simulink model "ElbowMusculoSkeletalModel"  (R2022b)
settings: Solver=FixedStepAuto  StartTime=0.0  StopTime=10  FixedStep=tstep  RelTol=1e-3
model workspace: external: MATLAB File C:\Users\hp\Desktop\Study\RAS MAE\EEE587\Project\ActivationDynamicsParameters.m (data not in the file)
values from neighbouring files (symbols this model uses):
  a0 = 0.286    [AllMuscleParams.m]    (also in equations.m)
  a1e = -0.014    [AllMuscleParams.m]    (also in equations.m)
  a2e = -3.96e-3    (= -0.00396)    [AllMuscleParams.m]    (also in equations.m)
  arel = 0.41    [AllMuscleParams.m]    (also in equations.m)
  brel = 5.2    [AllMuscleParams.m]    (also in equations.m)
  c = 1.373e-4    (= 0.0001373)    [AllMuscleParams.m]    (also in equations.m)
  Fmax = 1420    [AllMuscleParams.m]    (also in equations.m)
  Iarm = Marm*(Llarm^2)/3    (= 0.208333333333)    [AllMuscleParams.m]    (also in equations.m = Marm*(Llarm^2)/3)
  k = 2.90    (= 2.9)    [AllMuscleParams.m]    (also in equations.m)
  kpe = (0.5*Fmax)/(1 + width - (lpe_0/lce_opt))    (= 2730.76923077)    [AllMuscleParams.m]
  kse = Fmax/((0.04*lse_0)^2)    (= 29999323.9589)    [AllMuscleParams.m]    (also in equations.m = Fmax/((0.04*lse_0)^2))
  lce_init = lmtc_init-lse_0    (= 0.114)    [AllMuscleParams.m]
  lce_opt = 0.092    [AllMuscleParams.m]    (also in equations.m)
  Llarm = 0.5    [AllMuscleParams.m]    (also in equations.m)
  lpe_0 = 1.4*lce_opt    (= 0.1288)    [AllMuscleParams.m]
  lse_0 = 0.172    [AllMuscleParams.m]    (also in equations.m)
  m = 11.25    [AllMuscleParams.m]    (also in equations.m)
  Marm = 2.5    [AllMuscleParams.m]    (also in equations.m)
  q0 = 0.005    [AllMuscleParams.m]    (also in equations.m)
  qcrit = 0.03    [AllMuscleParams.m]
  ThetaInit = 0    [AllMuscleParams.m]
undefined symbols (not defined in the file or in its folder): DiscIntNeverNeededParam
libraries: simulink x2
settings Model: Creator=hp  LastModifiedBy=hp

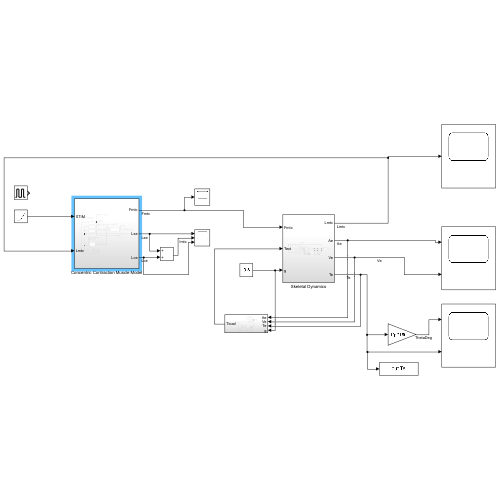
[thumbnail: Simulink's stored preview of the top-level diagram]
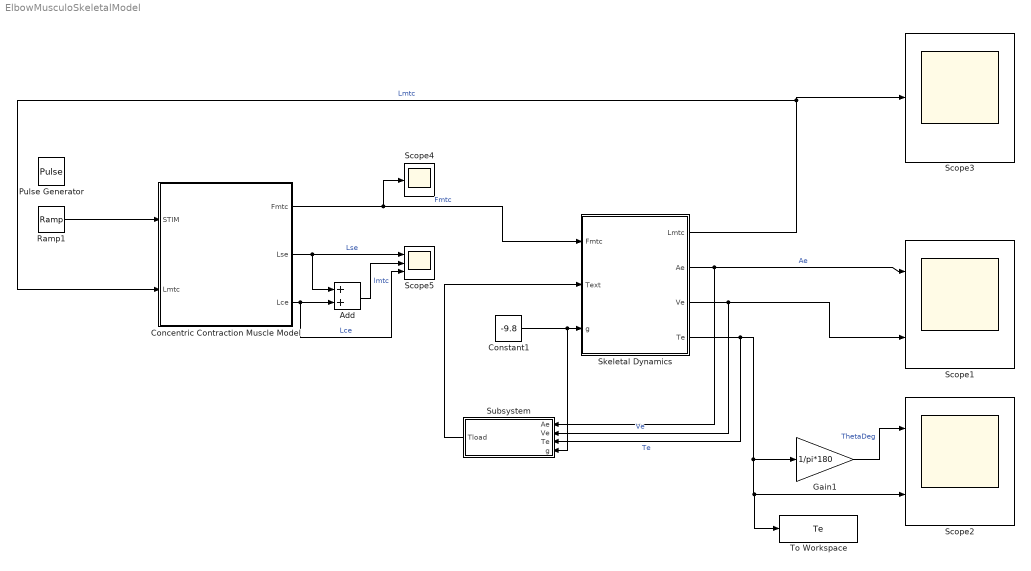
== system ElbowMusculoSkeletalModel ==
  Add : Sum
  Concentric Contraction Muscle Model : Subsystem
  Constant1 : Constant  Value=-9.8
  Gain1 : Gain  Gain=1/pi*180
  Pulse Generator : DiscretePulseGenerator  PulseType=Time based  Amplitude=10  Period=0.01  PulseWidth=50
  Ramp1 : simulink/Sources/Ramp  slope=0  start=0  InitialOutput=0.1
  Scope1 : Scope  NumInputPorts=2
  Scope2 : Scope  NumInputPorts=2
  Scope3 : Scope
  Scope4 : Scope
  Scope5 : Scope  NumInputPorts=3
  Skeletal Dynamics : Subsystem
  Subsystem : Subsystem
  To Workspace : ToWorkspace  VariableName=Te  SaveFormat=Timeseries  SampleTime=-1
  wires:
  Constant1/1 -> Subsystem/4(g), Skeletal Dynamics/3(g)
  Skeletal Dynamics/3(Ve) -> Subsystem/2(Ve), Scope1/2  "Ve"
  Skeletal Dynamics/4(Te) -> Subsystem/3(Te), To Workspace/1, Scope2/2, Gain1/1  "Te"
  Gain1/1 -> Scope2/1  "ThetaDeg"
  Skeletal Dynamics/2(Ae) -> Subsystem/1(Ae), Scope1/1  "Ae"
  Skeletal Dynamics/1(Lmtc) -> Concentric Contraction Muscle Model/2(Lmtc), Scope3/1  "Lmtc"
  Concentric Contraction Muscle Model/1(Fmtc) -> Skeletal Dynamics/1(Fmtc), Scope4/1  "Fmtc"
  Concentric Contraction Muscle Model/2(Lse) -> Add/1, Scope5/1  "Lse"
  Concentric Contraction Muscle Model/3(Lce) -> Add/2, Scope5/3  "Lce"
  Add/1 -> Scope5/2  "lmtc"
  Subsystem/1(Tload) -> Skeletal Dynamics/2(Text)
  Ramp1/1 -> Concentric Contraction Muscle Model/1(STIM)

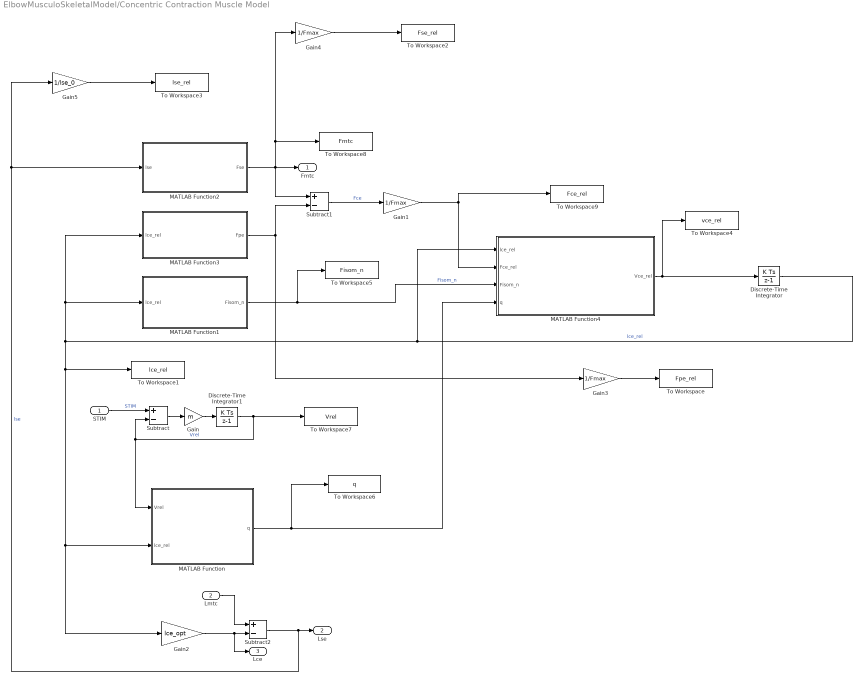
== system ElbowMusculoSkeletalModel/Concentric Contraction Muscle Model ==
  STIM : Inport
  Lmtc : Inport  Port=2
  Discrete-Time Integrator : DiscreteIntegrator  InitialCondition=lce_init/lce_opt  SampleTime=-1  ICPrevOutput=DiscIntNeverNeededParam  ICPrevScaledInput=DiscIntNeverNeededParam
  Discrete-Time Integrator1 : DiscreteIntegrator  SampleTime=-1  ICPrevOutput=DiscIntNeverNeededParam  ICPrevScaledInput=DiscIntNeverNeededParam
  Gain : Gain  Gain=m
  Gain1 : Gain  Gain=1/Fmax
  Gain2 : Gain  Gain=lce_opt
  Gain3 : Gain  Gain=1/Fmax
  Gain4 : Gain  Gain=1/Fmax
  Gain5 : Gain  Gain=1/lse_0
  MATLAB Function : MATLAB Function  TreatAsAtomicUnit=on
  MATLAB Function1 : MATLAB Function  TreatAsAtomicUnit=on
  MATLAB Function2 : MATLAB Function  TreatAsAtomicUnit=on
  MATLAB Function3 : MATLAB Function  TreatAsAtomicUnit=on
  MATLAB Function4 : MATLAB Function  TreatAsAtomicUnit=on
  Subtract : Sum  Inputs=+-
  Subtract1 : Sum  Inputs=+-
  Subtract2 : Sum  Inputs=+-
  To Workspace : ToWorkspace  VariableName=Fpe_rel  SaveFormat=Timeseries  SampleTime=-1
  To Workspace1 : ToWorkspace  VariableName=lce_rel  SaveFormat=Timeseries  SampleTime=-1
  To Workspace2 : ToWorkspace  VariableName=Fse_rel  SaveFormat=Timeseries  SampleTime=-1
  To Workspace3 : ToWorkspace  VariableName=lse_rel  SaveFormat=Timeseries  SampleTime=-1
  To Workspace4 : ToWorkspace  VariableName=vce_rel  SaveFormat=Timeseries  SampleTime=-1
  To Workspace5 : ToWorkspace  VariableName=Fisom_n  SaveFormat=Timeseries  SampleTime=-1
  To Workspace6 : ToWorkspace  VariableName=q  SaveFormat=Timeseries  SampleTime=-1
  To Workspace7 : ToWorkspace  VariableName=Vrel  SaveFormat=Timeseries  SampleTime=-1
  To Workspace8 : ToWorkspace  VariableName=Fmtc  SaveFormat=Timeseries  SampleTime=-1
  To Workspace9 : ToWorkspace  VariableName=Fce_rel  SaveFormat=Timeseries  SampleTime=-1
  Fmtc : Outport
  Lse : Outport  Port=2
  Lce : Outport  Port=3
  wires:
  Gain1/1 -> MATLAB Function4/2(Fce_rel), To Workspace9/1
  Discrete-Time Integrator1/1 -> To Workspace7/1, Subtract/2, MATLAB Function/1(Vrel)  "Vrel"
  MATLAB Function2/1(Fse) -> To Workspace8/1, Gain4/1, Fmtc/1, Subtract1/1
  Subtract/1 -> Gain/1
  MATLAB Function3/1(Fpe) -> Gain3/1, Subtract1/2
  STIM/1 -> Subtract/1  "STIM"
  Gain/1 -> Discrete-Time Integrator1/1
  Subtract2/1 -> Lse/1, Gain5/1, MATLAB Function2/1(lse)  "lse"
  MATLAB Function1/1(Fisom_n) -> To Workspace5/1, MATLAB Function4/3(Fisom_n)  "Fisom_n"
  MATLAB Function4/1(Vce_rel) -> To Workspace4/1, Discrete-Time Integrator/1
  Lmtc/1 -> Subtract2/1
  Subtract1/1 -> Gain1/1  "Fce"
  MATLAB Function/1(q) -> To Workspace6/1, MATLAB Function4/4(q)
  Gain3/1 -> To Workspace/1
  Gain5/1 -> To Workspace3/1
  Gain4/1 -> To Workspace2/1
  Gain2/1 -> Lce/1, Subtract2/2
  Discrete-Time Integrator/1 -> MATLAB Function4/1(lce_rel), MATLAB Function3/1(lce_rel), MATLAB Function1/1(lce_rel), To Workspace1/1, MATLAB Function/2(lce_rel), Gain2/1  "lce_rel"

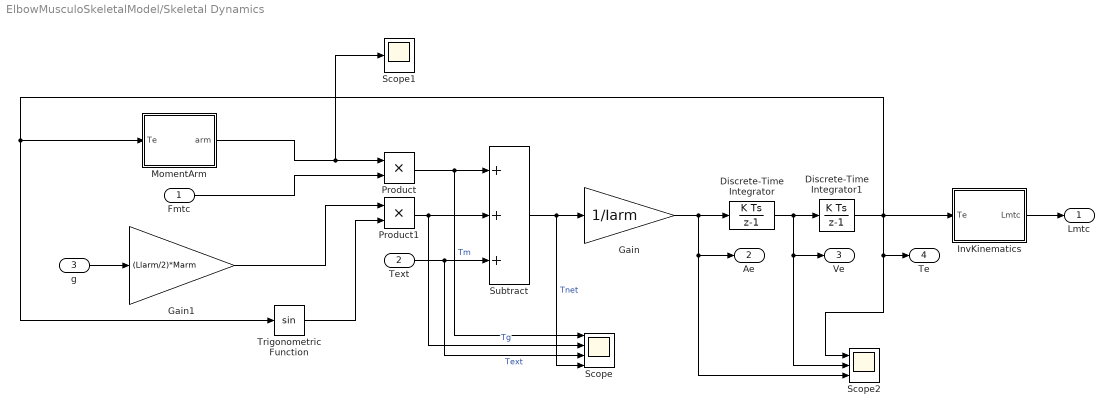
== system ElbowMusculoSkeletalModel/Skeletal Dynamics ==
  Fmtc : Inport
  Text : Inport  Port=2
  g : Inport  Port=3
  Discrete-Time Integrator : DiscreteIntegrator  SampleTime=-1  ICPrevOutput=DiscIntNeverNeededParam  ICPrevScaledInput=DiscIntNeverNeededParam
  Discrete-Time Integrator1 : DiscreteIntegrator  InitialCondition=ThetaInit  SampleTime=-1  ICPrevOutput=DiscIntNeverNeededParam  ICPrevScaledInput=DiscIntNeverNeededParam
  Gain : Gain  Gain=1/Iarm
  Gain1 : Gain  Gain=(Llarm/2)*Marm
  InvKinematics : MATLAB Function  TreatAsAtomicUnit=on
  MomentArm : MATLAB Function  TreatAsAtomicUnit=on
  Product : Product
  Product1 : Product
  Scope : Scope  NumInputPorts=4
  Scope1 : Scope
  Scope2 : Scope  NumInputPorts=3
  Subtract : Sum  Inputs=+++
  Trigonometric Function : Trigonometry
  Lmtc : Outport
  Ae : Outport  Port=2
  Ve : Outport  Port=3
  Te : Outport  Port=4
  wires:
  MomentArm/1(arm) -> Scope1/1, Product/1
  Fmtc/1 -> Product/2
  Discrete-Time Integrator/1 -> Scope2/2, Ve/1, Discrete-Time Integrator1/1
  Text/1 -> Scope/3, Subtract/3  "Text"
  Gain1/1 -> Product1/1
  g/1 -> Gain1/1
  Product1/1 -> Scope/2, Subtract/2  "Tg"
  Product/1 -> Scope/1, Subtract/1  "Tm"
  Trigonometric Function/1 -> Product1/2
  Subtract/1 -> Scope/4, Gain/1  "Tnet"
  Gain/1 -> Scope2/3, Ae/1, Discrete-Time Integrator/1
  Discrete-Time Integrator1/1 -> Scope2/1, Te/1, InvKinematics/1(Te), MomentArm/1(Te), Trigonometric Function/1
  InvKinematics/1(Lmtc) -> Lmtc/1

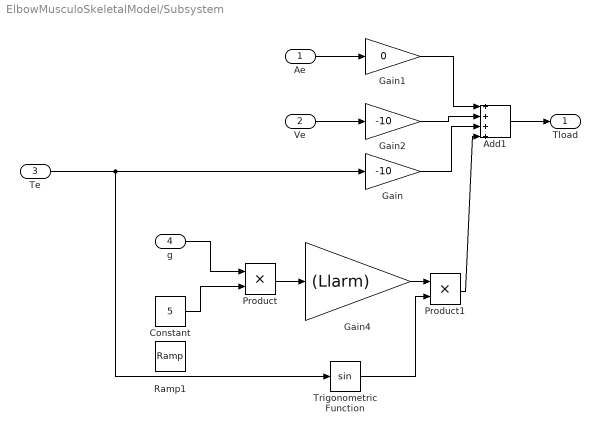
== system ElbowMusculoSkeletalModel/Subsystem ==
  Ae : Inport
  Ve : Inport  Port=2
  Te : Inport  Port=3
  g : Inport  Port=4
  Add1 : Sum  Inputs=++++
  Constant : Constant  Value=5
  Gain : Gain  Gain=-10
  Gain1 : Gain  Gain=0
  Gain2 : Gain  Gain=-10
  Gain4 : Gain  Gain=(Llarm)
  Product : Product
  Product1 : Product
  Ramp1 : simulink/Sources/Ramp  slope=5  start=5  InitialOutput=0
  Trigonometric Function : Trigonometry
  Tload : Outport
  wires:
  Add1/1 -> Tload/1
  Ve/1 -> Gain2/1
  Ae/1 -> Gain1/1
  Gain1/1 -> Add1/1
  Gain/1 -> Add1/3
  Gain2/1 -> Add1/2
  Te/1 -> Gain/1, Trigonometric Function/1
  g/1 -> Product/1
  Product/1 -> Gain4/1
  Gain4/1 -> Product1/1
  Trigonometric Function/1 -> Product1/2
  Product1/1 -> Add1/4
  Constant/1 -> Product/2

== matlab function ElbowMusculoSkeletalModel/Concentric Contraction Muscle Model/MATLAB Function1 ==
  data: lce_rel input; Fisom_n output; a parameter
function Fisom_n = ForceLengthFactor(lce_rel, a)

% h2
Fisom_n = -a*(lce_rel^2) + 2*a*lce_rel - a + 1;

== matlab function ElbowMusculoSkeletalModel/Concentric Contraction Muscle Model/MATLAB Function ==
  data: Vrel input; q output; k parameter; lce_rel input; q0 parameter; u parameter; c parameter
function q = ActivationDynamicsBlock(Vrel, k, lce_rel, q0, u, c)

% h3
rho = c*u*(k-1)/(k-lce_rel)*lce_rel;

% h1
q = (q0 + (rho*Vrel)^3)/(1 + (rho*Vrel)^3);

== matlab function ElbowMusculoSkeletalModel/Concentric Contraction Muscle Model/MATLAB Function2 ==
  data: lse input; Fse output; lse_0 parameter; kse parameter
function Fse = SeriesElasticForce(lse, lse_0, kse)

%Fse = max(0, kse*(lse-lse_0)^2);
Fse = kse*(lse-lse_0)^2;

== matlab function ElbowMusculoSkeletalModel/Concentric Contraction Muscle Model/MATLAB Function3 ==
  data: Fpe output; lce_rel input; kpe parameter; lce_opt parameter; lpe_0 parameter
function Fpe = ParallelElasticForce(lce_rel, kpe, lce_opt, lpe_0)

%Fpe = max(0, kpe*(lce_rel-(lpe_0/lce_opt))^2);
Fpe = 0;

== matlab function ElbowMusculoSkeletalModel/Concentric Contraction Muscle Model/MATLAB Function4 ==
  data: lce_rel input; Fce_rel input; Fisom_n input; Vce_rel output; q input; qcrit parameter; q0 parameter; brel parameter; arel parameter
function Vce_rel= ConcentricForceVelocityInverseFunc(lce_rel, Fce_rel, Fisom_n, q, qcrit, q0, brel, arel)

A = 1/(1+exp(-100*(lce_rel-1)));
B = 1/(1+exp(100*(lce_rel-1)));
arel_dot = arel*Fisom_n*(B*(1/Fisom_n) + A);
brel_dot = brel;

Vce_rel = brel_dot*(Fce_rel - q*Fisom_n)/(Fce_rel + q*arel_dot); % arel_dot assumed to be constant, independent of lce_rel

== matlab function ElbowMusculoSkeletalModel/Skeletal Dynamics/MomentArm ==
  data: arm output; Te input; a1e parameter; a2e parameter
function arm = fcn(Te, a1e, a2e)

%arm = a1e + 2*a2e*Te;
arm = -a1e;

== matlab function ElbowMusculoSkeletalModel/Skeletal Dynamics/InvKinematics ==
  data: Te input; Lmtc output; a0 parameter; a1e parameter; a2e parameter
function Lmtc = fcn(Te, a0, a1e, a2e)

Lmtc = a0 + (a1e*Te) + (a2e*(Te^2));
